simulink model "unicycle_with_odoloc"  (Simulink 8.9)
settings: Solver=ode45  StartTime=0.0  StopTime=T  MaxStep=0.01  RelTol=1e-3  EnableMultiTasking=on
values from neighbouring files (symbols this model uses):
  flag = 1    [init.m]
  freq = 1    [init.m]
  k_om = 0    [init.m]
  k_v = 0    [init.m]
  omega_bar = 1    [init.m]
  T_s = 0.1    [init.m]
  theta_0 = pi/2    (= 1.57079632679)    [init.m]
  v_bar = 10    [init.m]
  x_0 = -1    [init.m]
  y_0 = -2    [init.m]
settings Model: SuppressorTable=22 serialization::archive 11 0 6 0 0 0 0 0  Creator=marilena  LastModifiedBy=giuseppe  ExtModeAutoUpdateStatusClock=off
settings OptimizationCC: ExpressionDepthLimit=2147483647
settings DebuggingCC: SaveWithParameterizedLinksMsg=none  SolverPrmCheckMsg=warning
settings HardwareCC: TargetHWDeviceType=32-bit Generic
settings GRTTargetCC: TargetFcnLib=ansi_tfl_tmw.mat  GeneratePreprocessorConditionals=Use local settings

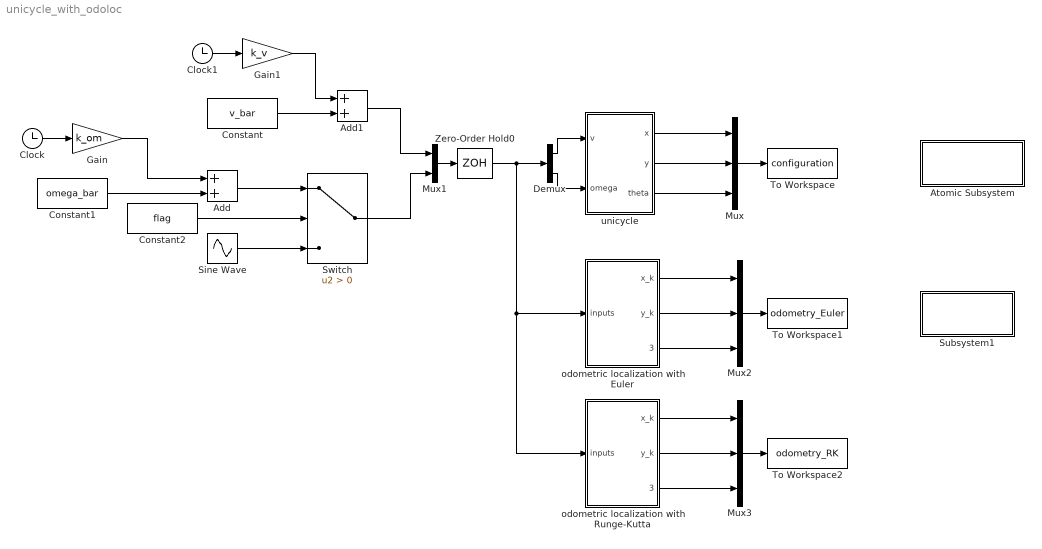
== system unicycle_with_odoloc ==
  Add : Sum
  Add1 : Sum
  Atomic Subsystem : Subsystem  TreatAsAtomicUnit=on
      settings: OpenFcn=init
      mask Display: disp('initialization')
  Clock : Clock
  Clock1 : Clock
  Constant : Constant  Value=v_bar
  Constant1 : Constant  Value=omega_bar
  Constant2 : Constant  Value=flag
  Demux : Demux  Outputs=2
  Gain : Gain  Gain=k_om
  Gain1 : Gain  Gain=k_v
  Mux : Mux  Inputs=3
  Mux1 : Mux  Inputs=2
  Mux2 : Mux  Inputs=3
  Mux3 : Mux  Inputs=3
  Sine Wave : Sin  Amplitude=omega_bar  Frequency=freq  SampleTime=0
  Subsystem1 : Subsystem
      settings: OpenFcn=plots
      mask Display: disp('plots')
  Switch : Switch  Criteria=u2 > Threshold
  To Workspace : ToWorkspace  VariableName=configuration  SaveFormat=Structure With Time
  To Workspace1 : ToWorkspace  VariableName=odometry_Euler  SaveFormat=Structure With Time
  To Workspace2 : ToWorkspace  VariableName=odometry_RK  SaveFormat=Structure With Time
  Zero-Order Hold0 : ZeroOrderHold  SampleTime=T_s
  odometric localization with Euler : Subsystem
  odometric localization with Runge-Kutta : Subsystem
  unicycle : Subsystem
  wires:
  Mux/1 -> To Workspace/1
  unicycle/3(theta) -> Mux/3
  unicycle/1(x) -> Mux/1
  unicycle/2(y) -> Mux/2
  Demux/1 -> unicycle/1(v)
  Demux/2 -> unicycle/2(omega)
  odometric localization with Euler/1(x_k) -> Mux2/1
  odometric localization with Euler/2(y_k) -> Mux2/2
  odometric localization with Euler/3(theta_k) -> Mux2/3
  Sine Wave/1 -> Switch/3
  Constant2/1 -> Switch/2
  Switch/1 -> Mux1/2
  odometric localization with Runge-Kutta/1(x_k) -> Mux3/1
  odometric localization with Runge-Kutta/2(y_k) -> Mux3/2
  odometric localization with Runge-Kutta/3(theta_k) -> Mux3/3
  Mux3/1 -> To Workspace2/1
  Mux2/1 -> To Workspace1/1
  Mux1/1 -> Zero-Order Hold0/1
  Zero-Order Hold0/1 -> odometric localization with Runge-Kutta/1(inputs), odometric localization with Euler/1(inputs), Demux/1
  Constant1/1 -> Add/2
  Clock/1 -> Gain/1
  Gain/1 -> Add/1
  Add/1 -> Switch/1
  Constant/1 -> Add1/2
  Add1/1 -> Mux1/1
  Clock1/1 -> Gain1/1
  Gain1/1 -> Add1/1

== system unicycle_with_odoloc/Atomic Subsystem ==

== system unicycle_with_odoloc/Subsystem1 ==

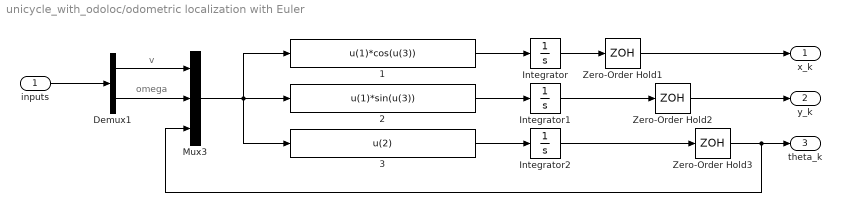
== system unicycle_with_odoloc/odometric localization with Euler ==
  note: omega
  note: v
  inputs : Inport
  " 1" : Fcn  Expr=u(1)*cos(u(3))
  " 2" : Fcn  Expr=u(1)*sin(u(3))
  " 3" : Fcn  Expr=u(2)
  Demux1 : Demux  Outputs=2
  Integrator : Integrator  InitialCondition=x_0
  Integrator1 : Integrator  InitialCondition=y_0
  Integrator2 : Integrator  InitialCondition=theta_0
  Mux3 : Mux  Inputs=3
  Zero-Order Hold1 : ZeroOrderHold  SampleTime=T_s
  Zero-Order Hold2 : ZeroOrderHold  SampleTime=T_s
  Zero-Order Hold3 : ZeroOrderHold  SampleTime=T_s
  x_k : Outport
  y_k : Outport  Port=2
  theta_k : Outport  Port=3
  wires:
  " 1"/1 -> Integrator/1
  " 2"/1 -> Integrator1/1
  Mux3/1 -> " 3"/1, " 1"/1, " 2"/1
  " 3"/1 -> Integrator2/1
  Integrator/1 -> Zero-Order Hold1/1
  Integrator1/1 -> Zero-Order Hold2/1
  Integrator2/1 -> Zero-Order Hold3/1
  Zero-Order Hold3/1 -> Mux3/3, theta_k/1
  Zero-Order Hold2/1 -> y_k/1
  Zero-Order Hold1/1 -> x_k/1
  Demux1/1 -> Mux3/1
  Demux1/2 -> Mux3/2
  inputs/1 -> Demux1/1

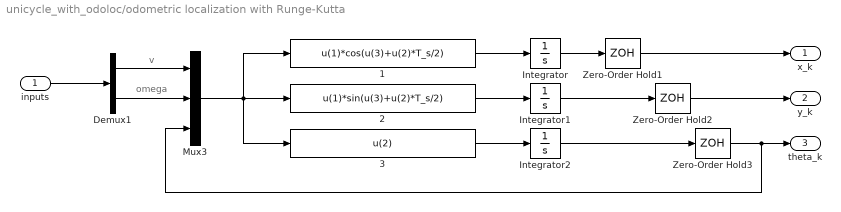
== system unicycle_with_odoloc/odometric localization with Runge-Kutta ==
  note: omega
  note: v
  inputs : Inport
  " 1" : Fcn  Expr=u(1)*cos(u(3)+u(2)*T_s/2)
  " 2" : Fcn  Expr=u(1)*sin(u(3)+u(2)*T_s/2)
  " 3" : Fcn  Expr=u(2)
  Demux1 : Demux  Outputs=2
  Integrator : Integrator  InitialCondition=x_0
  Integrator1 : Integrator  InitialCondition=y_0
  Integrator2 : Integrator  InitialCondition=theta_0
  Mux3 : Mux  Inputs=3
  Zero-Order Hold1 : ZeroOrderHold  SampleTime=T_s
  Zero-Order Hold2 : ZeroOrderHold  SampleTime=T_s
  Zero-Order Hold3 : ZeroOrderHold  SampleTime=T_s
  x_k : Outport
  y_k : Outport  Port=2
  theta_k : Outport  Port=3
  wires:
  " 1"/1 -> Integrator/1
  " 2"/1 -> Integrator1/1
  Mux3/1 -> " 3"/1, " 1"/1, " 2"/1
  " 3"/1 -> Integrator2/1
  Integrator/1 -> Zero-Order Hold1/1
  Integrator1/1 -> Zero-Order Hold2/1
  Integrator2/1 -> Zero-Order Hold3/1
  Zero-Order Hold3/1 -> Mux3/3, theta_k/1
  Zero-Order Hold2/1 -> y_k/1
  Zero-Order Hold1/1 -> x_k/1
  Demux1/1 -> Mux3/1
  Demux1/2 -> Mux3/2
  inputs/1 -> Demux1/1

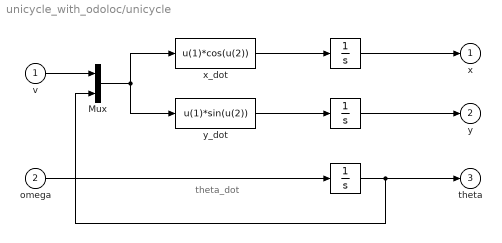
== system unicycle_with_odoloc/unicycle ==
  note: theta_dot
  v : Inport
  omega : Inport  Port=2
  " " : Integrator  InitialCondition=theta_0
  "   " : Integrator  InitialCondition=x_0
  "    " : Integrator  InitialCondition=y_0
  Mux : Mux  Inputs=2
  x_dot : Fcn  Expr=u(1)*cos(u(2))
  y_dot : Fcn  Expr=u(1)*sin(u(2))
  x : Outport
  y : Outport  Port=2
  theta : Outport  Port=3
  wires:
  v/1 -> Mux/1
  omega/1 -> " "/1
  x_dot/1 -> "   "/1
  y_dot/1 -> "    "/1
  " "/1 -> Mux/2, theta/1
  Mux/1 -> x_dot/1, y_dot/1
  "   "/1 -> x/1
  "    "/1 -> y/1
